simulink subsystem "MR_BladePitch_model"  (R2025a)
settings: Solver=VariableStepAuto  StartTime=0.0  StopTime=10.0  RelTol=1e-3
settings Model: Creator=Admin  LastModifiedBy=Admin

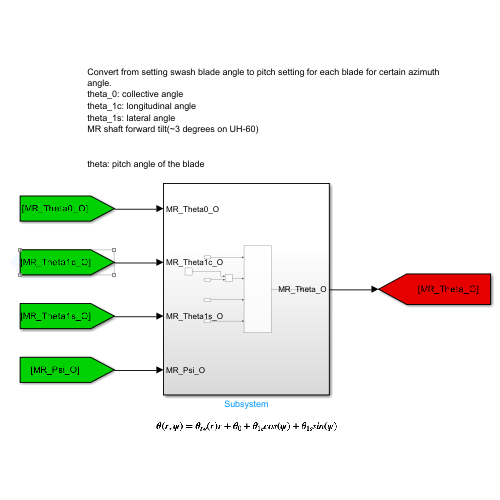
[thumbnail: Simulink's stored preview of the top-level diagram]
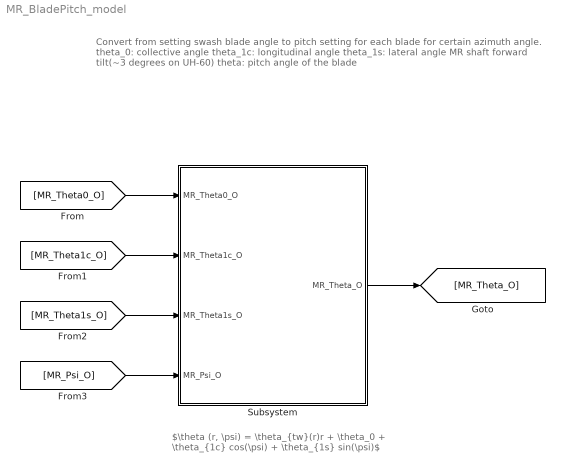
== system MR_BladePitch_model ==
  note: $\theta (r, \psi) = \theta_{tw}(r)r + \theta_0 + \theta_{1c} cos(\psi) + \theta_{1s} sin(\psi)$
  note: Convert from setting swash blade angle to pitch setting for each blade for certain azimuth angle.
      | theta_0: collective angle
      | theta_1c: longitudinal angle
      | theta_1s: lateral angle
      | MR shaft forward tilt(~3 degrees on UH-60)
      |
      | theta: pitch angle of the blade
  Subsystem : Subsystem
  wires:
  [MR_Theta0_O] -> Subsystem/1(MR_Theta0_O)
  [MR_Theta1c_O] -> Subsystem/2(MR_Theta1c_O)
  [MR_Theta1s_O] -> Subsystem/3(MR_Theta1s_O)
  [MR_Psi_O] -> Subsystem/4(MR_Psi_O)
  Subsystem/1(MR_Theta_O) -> [MR_Theta_O]

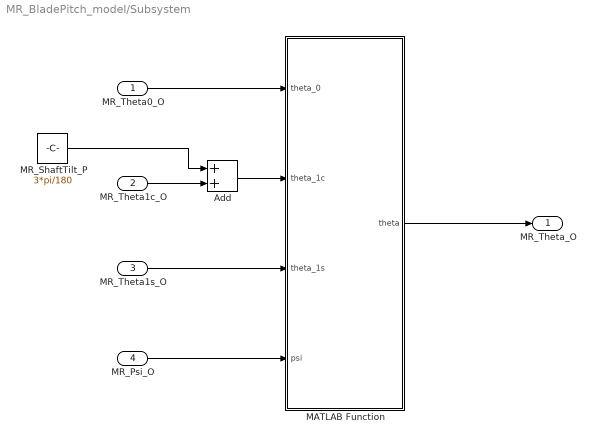
== system MR_BladePitch_model/Subsystem ==
  MR_Theta0_O : Inport
  MR_Theta1c_O : Inport  Port=2
  MR_Theta1s_O : Inport  Port=3
  MR_Psi_O : Inport  Port=4
  Add : Sum
  MATLAB Function : MATLAB Function  TreatAsAtomicUnit=on
  MR_ShaftTilt_P : Constant  Value=3*pi/180
  MR_Theta_O : Outport
  wires:
  MR_Theta1s_O/1 -> MATLAB Function/3(theta_1s)
  MATLAB Function/1(theta) -> MR_Theta_O/1
  Add/1 -> MATLAB Function/2(theta_1c)
  MR_ShaftTilt_P/1 -> Add/1
  MR_Theta0_O/1 -> MATLAB Function/1(theta_0)
  MR_Psi_O/1 -> MATLAB Function/4(psi)
  MR_Theta1c_O/1 -> Add/2

== matlab function MR_BladePitch_model/Subsystem/MATLAB Function ==
  data: theta_0 input; theta output; theta_1c input; theta_1s input; psi input
function theta = fcn(theta_0, theta_1c, theta_1s, psi)
theta_long = theta_1c * cos(psi);
theta_lat = theta_1s * sin(psi);

theta = theta_0 + theta_long + theta_lat;
